simulink model "lab2_sinusoidal_input"  (R2020b)
settings: Solver=FixedStepAuto  StartTime=0.0  StopTime=duration  FixedStep=0.01  RelTol=1e-3
values from neighbouring files (symbols this model uses):
  angular_frequency = frequencies(i)    [LabWork2.m]    (also in workspace.mat = 100)
  k = 14.4844    [workspace.mat]
  p = 190    [workspace.mat]
  tau = 0.191    [LabWork2.m]    (also in workspace.mat)
  z = 48    [workspace.mat]
settings Model: Creator=MSI  LastModifiedBy=berksahin

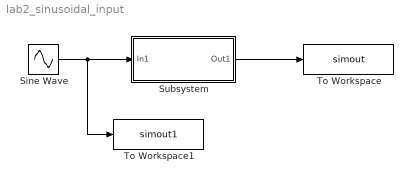
== system lab2_sinusoidal_input ==
  Sine Wave : Sin  Amplitude=10  Frequency=angular_frequency  SampleTime=0
  Subsystem : Subsystem
  To Workspace : ToWorkspace  VariableName=simout  SaveFormat=Timeseries  SampleTime=-1
  To Workspace1 : ToWorkspace  VariableName=simout1  SaveFormat=Timeseries  SampleTime=-1
  wires:
  Subsystem/1(Out1) -> To Workspace/1
  Sine Wave/1 -> To Workspace1/1, Subsystem/1(In1)

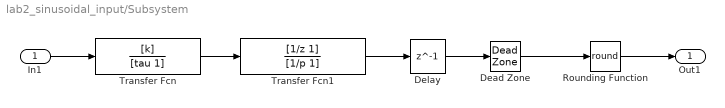
== system lab2_sinusoidal_input/Subsystem ==
  In1 : Inport
  Dead Zone : DeadZone  LowerValue=-5  UpperValue=5  SaturateOnIntegerOverflow=on
  Delay : Delay  DelayLength=1
  Rounding Function : Rounding  Operator=round
  Transfer Fcn : TransferFcn  Numerator=[k]  Denominator=[tau 1]
  Transfer Fcn1 : TransferFcn  Numerator=[1/z 1]  Denominator=[1/p 1]
  Out1 : Outport
  wires:
  Transfer Fcn/1 -> Transfer Fcn1/1
  In1/1 -> Transfer Fcn/1
  Rounding Function/1 -> Out1/1
  Delay/1 -> Dead Zone/1
  Transfer Fcn1/1 -> Delay/1
  Dead Zone/1 -> Rounding Function/1
